simulink model "Task_No6"  (R2023b)
settings: Solver=ode5  StartTime=0.0  StopTime=3600*24*7  FixedStep=1  RelTol=1e-3
InitFcn:
  | PARAMETERS;
StartFcn:
  | PARAMETERS;
values from neighbouring files (symbols this model uses):
  Conv_C_to_K = 273.15    [PARAMETERS.m]
  P_AC_AIR_FLOW = 1    [PARAMETERS.m]
  P_CP_AIR = 1012    [PARAMETERS.m]
  P_DENSITY_AIR = 1.2041    [PARAMETERS.m]
  P_DENSITY_BRICK = 2/(10^-3)    (= 2000)    [PARAMETERS.m]
  P_DENSITY_PUR = 150    [PARAMETERS.m]
  P_EM_GLASS = 0.94    [PARAMETERS.m]
  P_EM_WALL = 0.94    [PARAMETERS.m]
  P_HANDLER_AIR_FLOW = 0.1    [PARAMETERS.m]
  P_HUMAN = 100    [PARAMETERS.m]
  P_INIT_CO2 = 420    [PARAMETERS.m]
  P_M_HUMAN_CO2 = 0.02*P_DENSITY_CO2/3600    (= 1.1e-05)    [PARAMETERS.m]
  P_M_HUMAN_VAPOR = 500*10^-3/(24*3600)    (= 5.78703703704e-06)    [PARAMETERS.m]
  P_M_WINDOW_SPEC = 20    [PARAMETERS.m]
  P_THICK_BRICK = 0.175    [PARAMETERS.m]
  P_THICK_PUR = P_THICK_WALL - P_THICK_BRICK    (= 0.125)    [PARAMETERS.m]
  RH_INIT_BDR = 40    [PARAMETERS.m]
  T_BREATH = 34    [PARAMETERS.m]
  T_COOLER = 12    [PARAMETERS.m]
  T_HEATER = 50    [PARAMETERS.m]
  T_INIT_BDR = 22    [PARAMETERS.m]
  T_INIT_OUT = 2.9    [PARAMETERS.m]
  U_WALL = 0.32    [PARAMETERS.m]
  U_WINDOW = 3.0    (= 3)    [PARAMETERS.m]
undefined symbols (not defined in the file or in its folder): P_AREA_BATH, P_AREA_BDR1, P_AREA_BDR2, P_AREA_EAST_WALL_BATH, P_AREA_EAST_WALL_BDR2, P_AREA_EAST_WALL_KIT, P_AREA_HALL, P_AREA_KIT, P_AREA_LVR, P_AREA_NORTH_WALL_BATH, P_AREA_NORTH_WALL_BDR1, P_AREA_NORTH_WALL_BDR2, P_AREA_OUTER_WALL_BATH, P_AREA_OUTER_WALL_BDR1, P_AREA_OUTER_WALL_BDR2, P_AREA_OUTER_WALL_HALL, P_AREA_OUTER_WALL_KIT, P_AREA_OUTER_WALL_LVR, P_AREA_SOUTH_WALL_KIT, P_AREA_SOUTH_WALL_LVR, P_AREA_WALL_BATH_KIT, P_AREA_WALL_BDR1_BDR2, P_AREA_WALL_BDR1_HALL, P_AREA_WALL_BDR2_BATH, P_AREA_WALL_BDR2_HALL, P_AREA_WALL_HALL_BATH, P_AREA_WALL_HALL_LVR, P_AREA_WALL_LVR_KIT, P_AREA_WIN_BATH, P_AREA_WIN_BDRS, P_AREA_WIN_KIT, P_AREA_WIN_LVR, P_M_AIR_BATH, P_M_AIR_BDR1, P_M_AIR_BDR2, P_M_AIR_HALL, P_M_AIR_KIT, P_M_AIR_LVR, TBL_SOL_EAST_01, TBL_SOL_EAST_02, TBL_SOL_EAST_03, TBL_SOL_EAST_04, TBL_SOL_EAST_05, TBL_SOL_EAST_06, TBL_SOL_EAST_07, TBL_SOL_EAST_08, TBL_SOL_EAST_09, TBL_SOL_EAST_10, TBL_SOL_EAST_11, TBL_SOL_EAST_12, TBL_SOL_NORTH_01, TBL_SOL_NORTH_02, TBL_SOL_NORTH_03, TBL_SOL_NORTH_04, TBL_SOL_NORTH_05, TBL_SOL_NORTH_06, TBL_SOL_NORTH_07, TBL_SOL_NORTH_08, TBL_SOL_NORTH_09, TBL_SOL_NORTH_10 ... (+7)
libraries: fl_lib x166, nesl_utility x88, slpidlib x3
(part 4 of 5)

== system Task_No6/sub_House/Bedroom 2/Bedroom 2/Window (BDR2<->Outside) ==
  InAir-Window : fl_lib/Thermal/Thermal Elements/Thermal Resistance  resistance=1/(U_WINDOW*P_AREA_WIN_BDRS*2)/2 K/W  T_specify=off  T_priority=None  T=0 K  T_nominal_specify=off  T_nominal_unit=K  T_nominal_value=1  Q_specify=off  Q_priority=None  Q=0 W  Q_nominal_specify=off  Q_nominal_unit=W  Q_nominal_value=1
  Thermal Mass of window : fl_lib/Thermal/Thermal Elements/Thermal Mass  mass_type=foundation.enum.constant_variable.constant  mass=P_M_WINDOW_SPEC*P_AREA_WIN_BDRS*2 kg  sp_heat=P_CP_GLASS J/(K*kg)  mass_min=1e-6 kg  num_ports=foundation.enum.numPorts2.one  m_specify=off  m_priority=High  m=1 kg  m_nominal_specify=off  m_nominal_unit=kg  m_nominal_value=1  T_specify=on  T_priority=High  T=T_INIT_BDR degC  T_nominal_specify=off  T_nominal_unit=K  T_nominal_value=1  Q_specify=off  Q_priority=None  Q=0 W  Q_nominal_specify=off  Q_nominal_unit=W  Q_nominal_value=1
  Window-OutAir : fl_lib/Thermal/Thermal Elements/Thermal Resistance  resistance=1/(U_WINDOW*P_AREA_WIN_BDRS*2)/2 K/W  T_specify=off  T_priority=None  T=0 K  T_nominal_specify=off  T_nominal_unit=K  T_nominal_value=1  Q_specify=off  Q_priority=None  Q=0 W  Q_nominal_specify=off  Q_nominal_unit=W  Q_nominal_value=1
  Conn1 : PMIOPort  Side=Right
  Conn2 : PMIOPort  Port=2  Side=Left
  Conn3 : PMIOPort  Port=3  Side=Right
  connections:
  Conn2/RConn1 -- InAir-Window/LConn1
  Conn1/RConn1 -- Window-OutAir/RConn1
  InAir-Window/RConn1 -- Thermal Mass of window/LConn1 -- Conn3/RConn1 -- Window-OutAir/LConn1

== system Task_No6/sub_House/Bedroom 2/MA Bedroom 2/Environment_in ==
  Constant1 : Constant  Value=P_INIT_CO2
  Constant4 : Constant  Value=1e5
  Constant6 : Constant  Value=Conv_C_to_K
  Controlled Reservoir (MA) : fl_lib/Moist Air/Elements/Controlled Reservoir (MA)  moisture_spec=foundation.enum.moistureSpec.RelativeHumidity  trace_gas_spec=foundation.enum.trace_gas_spec.mass_fraction  RH_ws=1  area_A=P_AREA_DUCT m^2  input_error_spec=foundation.enum.input_range_error.warn
      settings: InternalSimscapePortConfiguration="{\"Bottom\":[],\"Left\":[{\"id\":\"A\",\"label\":\"A\",\"type\":\"foundation.moist_air.moist_air\"}],\"Right\":[{\"id\":\"T\",\"label\":\"T\",\"type\":\"input\"},{\"id\":\"P\",\"label\":\"P\",\"type\":\"input\"},{\"id\":\"W\",\"label\":\"W\",\"type\":\"input\"},{\"id\":\"G\",\"label\":\"G\",\"type\":\"input\"}],\"Top\":[]}"
  Gain : Gain  Gain=1/100
  Gain2 : Gain  Gain=1e-6
  Simulink-PS Converter{3,5..7} (4 alike) : nesl_utility/Simulink-PS Converter  PhysicalDomain=network_engine_domain  SubClassName=ps_input  LeftPortType=input  RightPortType=output  PseudoPeriodic=off  Frequencies=[]  NoiseDistribution=none  NoiseParameters=[]  Unit=1  AffineConversion=off  FilteringAndDerivatives=provide  SimscapeFilterOrder=1  InputFilterTimeConstant=0.001  UdotUserProvided=0
  Sum2 : Sum  Inputs=|++
  Conn1 : PMIOPort  Side=Left
  wires:
  Constant1/1 -> Gain2/1
  Constant6/1 -> Sum2/2
  Gain/1 -> Simulink-PS Converter6/1
  Constant4/1 -> Simulink-PS Converter5/1
  Gain2/1 -> Simulink-PS Converter7/1
  Sum2/1 -> Simulink-PS Converter3/1
  [T_OUT] -> Sum2/1
  [RH_OUT] -> Gain/1
  connections:
  Simulink-PS Converter3/RConn1 -- Controlled Reservoir (MA)/RConn1
  Simulink-PS Converter7/RConn1 -- Controlled Reservoir (MA)/RConn4
  Controlled Reservoir (MA)/LConn1 -- Conn1/RConn1
  Simulink-PS Converter5/RConn1 -- Controlled Reservoir (MA)/RConn2
  Simulink-PS Converter6/RConn1 -- Controlled Reservoir (MA)/RConn3

== system Task_No6/sub_House/Bedroom 2/MA Bedroom 2/Moisture & CO2 Gain ==
  Constant : Constant  Value=T_BREATH
  Constant1 : Constant  Value=P_M_HUMAN_VAPOR
  Constant2 : Constant  Value=P_M_HUMAN_CO2
  Constant3 : Constant  Value=Conv_C_to_K
  Inhabitant CO2 Gain : fl_lib/Moist Air/Sources/Moisture & Trace Gas Sources/Trace Gas Source (MA)  source_type=foundation.enum.constant_controlled.controlled  trace_gas_mass_flow=P_M_HUMAN_CO2 kg/s  temperature_spec=foundation.enum.temperature_spec.specified  trace_gas_temperature=T_BREATH degC  Phi_S_specify=off  Phi_S_priority=None  Phi_S=0 kW  Phi_S_nominal_specify=off  Phi_S_nominal_unit=kW  Phi_S_nominal_value=1  mdot_g_S_specify=off  mdot_g_S_priority=None  mdot_g_S=0 kg/s  mdot_g_S_nominal_specify=off  mdot_g_S_nominal_unit=kg/s  mdot_g_S_nominal_value=1
      settings: InternalSimscapePortConfiguration="{\"Bottom\":[],\"Left\":[{\"id\":\"S\",\"label\":\"S\",\"type\":\"foundation.moist_air.moist_air_source\"}],\"Right\":[{\"id\":\"M\",\"label\":\"M\",\"type\":\"input\"},{\"id\":\"T\",\"label\":\"T\",\"type\":\"input\"}],\"Top\":[]}"
  Inhabitant Moisture Gain : fl_lib/Moist Air/Sources/Moisture & Trace Gas Sources/Moisture Source (MA)  source_type=foundation.enum.constant_controlled.controlled  moisture_source_spec=foundation.enum.moisture_source_spec.vapor  moisture_mass_flow=P_M_HUMAN_VAPOR kg/s  temperature_spec=foundation.enum.temperature_spec.specified  moisture_temperature=T_BREATH degC  Phi_S_specify=off  Phi_S_priority=None  Phi_S=0 kW  Phi_S_nominal_specify=off  Phi_S_nominal_unit=kW  Phi_S_nominal_value=1  mdot_w_S_specify=off  mdot_w_S_priority=None  mdot_w_S=0 kg/s  mdot_w_S_nominal_specify=off  mdot_w_S_nominal_unit=kg/s  mdot_w_S_nominal_value=1
      settings: InternalSimscapePortConfiguration="{\"Bottom\":[],\"Left\":[{\"id\":\"S\",\"label\":\"S\",\"type\":\"foundation.moist_air.moist_air_source\"}],\"Right\":[{\"id\":\"M\",\"label\":\"M\",\"type\":\"input\"},{\"id\":\"T\",\"label\":\"T\",\"type\":\"input\"}],\"Top\":[]}"
  Product : Product
  Product1 : Product
  Simulink-PS Converter : nesl_utility/Simulink-PS Converter  PhysicalDomain=network_engine_domain  SubClassName=ps_input  LeftPortType=input  RightPortType=output  PseudoPeriodic=off  Frequencies=[]  NoiseDistribution=none  NoiseParameters=[]  Unit=1  AffineConversion=off  FilteringAndDerivatives=provide  SimscapeFilterOrder=1  InputFilterTimeConstant=0.001  UdotUserProvided=0
  Simulink-PS Converter1 : nesl_utility/Simulink-PS Converter  PhysicalDomain=network_engine_domain  SubClassName=ps_input  LeftPortType=input  RightPortType=output  PseudoPeriodic=off  Frequencies=[]  NoiseDistribution=none  NoiseParameters=[]  Unit=1  AffineConversion=off  FilteringAndDerivatives=provide  SimscapeFilterOrder=1  InputFilterTimeConstant=0.001  UdotUserProvided=0
  Simulink-PS Converter3 : nesl_utility/Simulink-PS Converter  PhysicalDomain=network_engine_domain  SubClassName=ps_input  LeftPortType=input  RightPortType=output  PseudoPeriodic=off  Frequencies=[]  NoiseDistribution=none  NoiseParameters=[]  Unit=1  AffineConversion=off  FilteringAndDerivatives=provide  SimscapeFilterOrder=1  InputFilterTimeConstant=0.001  UdotUserProvided=0
  Sum : Sum  Inputs=++|
  Conn1 : PMIOPort  Side=Left
  wires:
  Sum/1 -> Simulink-PS Converter1/1
  Product1/1 -> Simulink-PS Converter3/1
  Constant1/1 -> Product/2
  Constant/1 -> Sum/2
  Constant3/1 -> Sum/1
  [N_BDR2] -> Product/1
  Product/1 -> Simulink-PS Converter/1
  Constant2/1 -> Product1/2
  [N_BDR2] -> Product1/1
  connections:
  Simulink-PS Converter/RConn1 -- Inhabitant Moisture Gain/RConn1
  Simulink-PS Converter3/RConn1 -- Inhabitant CO2 Gain/RConn1
  Conn1/RConn1 -- Inhabitant Moisture Gain/LConn1 -- Inhabitant CO2 Gain/LConn1
  Inhabitant CO2 Gain/RConn2 -- Simulink-PS Converter1/RConn1 -- Inhabitant Moisture Gain/RConn2

== system Task_No6/sub_House/Hallway/Hallway/Ceiling & Floor (Hall<->Above & Below) ==
  Ceiling-InAir : fl_lib/Thermal/Thermal Elements/Thermal Resistance  resistance=1/(U_CEIL*P_AREA_HALL) K/W  T_specify=off  T_priority=None  T=0 K  T_nominal_specify=off  T_nominal_unit=K  T_nominal_value=1  Q_specify=off  Q_priority=None  Q=0 W  Q_nominal_specify=off  Q_nominal_unit=W  Q_nominal_value=1
  Floor-InAir : fl_lib/Thermal/Thermal Elements/Thermal Resistance  resistance=1/(U_CEIL*P_AREA_HALL) K/W  T_specify=off  T_priority=None  T=0 K  T_nominal_specify=off  T_nominal_unit=K  T_nominal_value=1  Q_specify=off  Q_priority=None  Q=0 W  Q_nominal_specify=off  Q_nominal_unit=W  Q_nominal_value=1
  Conn1 : PMIOPort  Side=Left
  Conn2 : PMIOPort  Port=2  Side=Right
  connections:
  Floor-InAir/RConn1 -- Ceiling-InAir/RConn1 -- Conn2/RConn1
  Floor-InAir/LConn1 -- Ceiling-InAir/LConn1 -- Conn1/RConn1

== system Task_No6/sub_House/Hallway/Hallway/Inside Enivornment Temperature ==
  T_ENV : Inport
  Constant2 : Constant  Value=Conv_C_to_K
  Controlled Temperature Source : fl_lib/Thermal/Thermal Sources/Controlled Temperature Source
  Simulink-PS Converter1 : nesl_utility/Simulink-PS Converter  PhysicalDomain=network_engine_domain  SubClassName=ps_input  LeftPortType=input  RightPortType=output  PseudoPeriodic=off  Frequencies=[]  NoiseDistribution=none  NoiseParameters=[]  Unit=1  AffineConversion=off  FilteringAndDerivatives=provide  SimscapeFilterOrder=1  InputFilterTimeConstant=0.001  UdotUserProvided=0
  Sum : Sum  Inputs=|++
  Thermal Reference1 : fl_lib/Thermal/Thermal Elements/Thermal Reference
  Conn1 : PMIOPort  Side=Left
  wires:
  T_ENV/1 -> Sum/1
  Constant2/1 -> Sum/2
  Sum/1 -> Simulink-PS Converter1/1
  connections:
  Controlled Temperature Source/LConn1 -- Conn1/RConn1
  Simulink-PS Converter1/RConn1 -- Controlled Temperature Source/RConn1
  Thermal Reference1/LConn1 -- Controlled Temperature Source/RConn2

== system Task_No6/sub_House/Hallway/Hallway/Outside Temperature ==
  T_OUT : Inport
  Constant2 : Constant  Value=Conv_C_to_K
  Controlled Temperature Source : fl_lib/Thermal/Thermal Sources/Controlled Temperature Source
  Simulink-PS Converter1 : nesl_utility/Simulink-PS Converter  PhysicalDomain=network_engine_domain  SubClassName=ps_input  LeftPortType=input  RightPortType=output  PseudoPeriodic=off  Frequencies=[]  NoiseDistribution=none  NoiseParameters=[]  Unit=1  AffineConversion=off  FilteringAndDerivatives=provide  SimscapeFilterOrder=1  InputFilterTimeConstant=0.001  UdotUserProvided=0
  Sum : Sum  Inputs=|++
  Thermal Reference1 : fl_lib/Thermal/Thermal Elements/Thermal Reference
  Conn1 : PMIOPort  Side=Left
  wires:
  Sum/1 -> Simulink-PS Converter1/1
  Constant2/1 -> Sum/2
  T_OUT/1 -> Sum/1
  connections:
  Thermal Reference1/LConn1 -- Controlled Temperature Source/RConn2
  Simulink-PS Converter1/RConn1 -- Controlled Temperature Source/RConn1
  Controlled Temperature Source/LConn1 -- Conn1/RConn1

== system Task_No6/sub_House/Hallway/Hallway/TEMP_01 ==
  Constant2 : Constant  Value=Conv_C_to_K
  PS-Simulink Converter : nesl_utility/PS-Simulink Converter  PhysicalDomain=network_engine_domain  SubClassName=ps_output  LeftPortType=input  RightPortType=output  PseudoPeriodic=off  Frequencies=[]  VectorFormat=inherit  Unit=inherit  AffineConversion=off
  Sum : Sum  Inputs=|+-
  Temperature Sensor : fl_lib/Thermal/Thermal Sensors/Temperature Sensor  temperature_measure=foundation.enum.MeasurementReference.difference
  Thermal Reference2 : fl_lib/Thermal/Thermal Elements/Thermal Reference
  PS : PMIOPort  Side=Left
  Sim : Outport
  wires:
  Sum/1 -> Sim/1
  PS-Simulink Converter/1 -> Sum/1
  Constant2/1 -> Sum/2
  connections:
  Thermal Reference2/LConn1 -- Temperature Sensor/RConn1
  PS-Simulink Converter/LConn1 -- Temperature Sensor/RConn2
  PS/RConn1 -- Temperature Sensor/LConn1

== system Task_No6/sub_House/Hallway/Hallway/Wall (Hall<->Outside) ==
  InAir-Wall : fl_lib/Thermal/Thermal Elements/Thermal Resistance  resistance=1/(U_WALL*P_AREA_OUTER_WALL_HALL)/2 K/W  T_specify=off  T_priority=None  T=0 K  T_nominal_specify=off  T_nominal_unit=K  T_nominal_value=1  Q_specify=off  Q_priority=None  Q=0 W  Q_nominal_specify=off  Q_nominal_unit=W  Q_nominal_value=1
  Thermal Mass of wall : fl_lib/Thermal/Thermal Elements/Thermal Mass  mass_type=foundation.enum.constant_variable.constant  mass=P_AREA_OUTER_WALL_HALL*(P_THICK_BRICK*P_DENSITY_BRICK+P_THICK_PUR*P_DENSITY_PUR) kg  sp_heat=P_CP_WALL J/(K*kg)  mass_min=1e-6 kg  num_ports=foundation.enum.numPorts2.one  m_specify=off  m_priority=High  m=1 kg  m_nominal_specify=off  m_nominal_unit=kg  m_nominal_value=1  T_specify=on  T_priority=High  T=T_INIT_BDR degC  T_nominal_specify=off  T_nominal_unit=K  T_nominal_value=1  Q_specify=off  Q_priority=None  Q=0 W  Q_nominal_specify=off  Q_nominal_unit=W  Q_nominal_value=1
  Wall-OutAir : fl_lib/Thermal/Thermal Elements/Thermal Resistance  resistance=1/(U_WALL*P_AREA_OUTER_WALL_HALL)/2 K/W  T_specify=off  T_priority=None  T=0 K  T_nominal_specify=off  T_nominal_unit=K  T_nominal_value=1  Q_specify=off  Q_priority=None  Q=0 W  Q_nominal_specify=off  Q_nominal_unit=W  Q_nominal_value=1
  Conn1 : PMIOPort  Side=Left
  Conn2 : PMIOPort  Port=2  Side=Right
  connections:
  Conn1/RConn1 -- InAir-Wall/LConn1
  InAir-Wall/RConn1 -- Thermal Mass of wall/LConn1 -- Wall-OutAir/LConn1
  Wall-OutAir/RConn1 -- Conn2/RConn1

== system Task_No6/sub_House/Kitchen/Kitchen/Ceiling & Floor (KIT<->Above & Below) ==
  Ceiling-InAir : fl_lib/Thermal/Thermal Elements/Thermal Resistance  resistance=1/(U_CEIL*P_AREA_KIT) K/W  T_specify=off  T_priority=None  T=0 K  T_nominal_specify=off  T_nominal_unit=K  T_nominal_value=1  Q_specify=off  Q_priority=None  Q=0 W  Q_nominal_specify=off  Q_nominal_unit=W  Q_nominal_value=1
  Floor-InAir : fl_lib/Thermal/Thermal Elements/Thermal Resistance  resistance=1/(U_CEIL*P_AREA_KIT) K/W  T_specify=off  T_priority=None  T=0 K  T_nominal_specify=off  T_nominal_unit=K  T_nominal_value=1  Q_specify=off  Q_priority=None  Q=0 W  Q_nominal_specify=off  Q_nominal_unit=W  Q_nominal_value=1
  Conn1 : PMIOPort  Side=Left
  Conn2 : PMIOPort  Port=2  Side=Right
  connections:
  Floor-InAir/RConn1 -- Ceiling-InAir/RConn1 -- Conn2/RConn1
  Floor-InAir/LConn1 -- Ceiling-InAir/LConn1 -- Conn1/RConn1

== system Task_No6/sub_House/Kitchen/Kitchen/Heat source human ==
  Constant : Constant  Value=P_HUMAN
  Controlled Heat Flow Rate Source : fl_lib/Thermal/Thermal Sources/Controlled Heat Flow Rate Source
  Product : Product
  Simulink-PS Converter : nesl_utility/Simulink-PS Converter  PhysicalDomain=network_engine_domain  SubClassName=ps_input  LeftPortType=input  RightPortType=output  PseudoPeriodic=off  Frequencies=[]  NoiseDistribution=none  NoiseParameters=[]  Unit=1  AffineConversion=off  FilteringAndDerivatives=provide  SimscapeFilterOrder=1  InputFilterTimeConstant=0.001  UdotUserProvided=0
  Thermal Reference : fl_lib/Thermal/Thermal Elements/Thermal Reference
  Conn1 : PMIOPort  Side=Left
  wires:
  [N_KIT] -> Product/1
  Constant/1 -> Product/2
  Product/1 -> Simulink-PS Converter/1
  connections:
  Thermal Reference/LConn1 -- Controlled Heat Flow Rate Source/RConn2
  Simulink-PS Converter/RConn1 -- Controlled Heat Flow Rate Source/RConn1
  Controlled Heat Flow Rate Source/LConn1 -- Conn1/RConn1

== system Task_No6/sub_House/Kitchen/Kitchen/Inside Enivornment Temperature ==
  T_ENV : Inport
  Constant2 : Constant  Value=Conv_C_to_K
  Controlled Temperature Source : fl_lib/Thermal/Thermal Sources/Controlled Temperature Source
  Simulink-PS Converter1 : nesl_utility/Simulink-PS Converter  PhysicalDomain=network_engine_domain  SubClassName=ps_input  LeftPortType=input  RightPortType=output  PseudoPeriodic=off  Frequencies=[]  NoiseDistribution=none  NoiseParameters=[]  Unit=1  AffineConversion=off  FilteringAndDerivatives=provide  SimscapeFilterOrder=1  InputFilterTimeConstant=0.001  UdotUserProvided=0
  Sum : Sum  Inputs=|++
  Thermal Reference1 : fl_lib/Thermal/Thermal Elements/Thermal Reference
  Conn1 : PMIOPort  Side=Left
  wires:
  T_ENV/1 -> Sum/1
  Constant2/1 -> Sum/2
  Sum/1 -> Simulink-PS Converter1/1
  connections:
  Controlled Temperature Source/LConn1 -- Conn1/RConn1
  Simulink-PS Converter1/RConn1 -- Controlled Temperature Source/RConn1
  Thermal Reference1/LConn1 -- Controlled Temperature Source/RConn2

== system Task_No6/sub_House/Kitchen/Kitchen/Outside Temperature ==
  T_OUT : Inport
  Constant2 : Constant  Value=Conv_C_to_K
  Controlled Temperature Source : fl_lib/Thermal/Thermal Sources/Controlled Temperature Source
  Simulink-PS Converter1 : nesl_utility/Simulink-PS Converter  PhysicalDomain=network_engine_domain  SubClassName=ps_input  LeftPortType=input  RightPortType=output  PseudoPeriodic=off  Frequencies=[]  NoiseDistribution=none  NoiseParameters=[]  Unit=1  AffineConversion=off  FilteringAndDerivatives=provide  SimscapeFilterOrder=1  InputFilterTimeConstant=0.001  UdotUserProvided=0
  Sum : Sum  Inputs=|++
  Thermal Reference1 : fl_lib/Thermal/Thermal Elements/Thermal Reference
  Conn1 : PMIOPort  Side=Left
  wires:
  Sum/1 -> Simulink-PS Converter1/1
  Constant2/1 -> Sum/2
  T_OUT/1 -> Sum/1
  connections:
  Thermal Reference1/LConn1 -- Controlled Temperature Source/RConn2
  Simulink-PS Converter1/RConn1 -- Controlled Temperature Source/RConn1
  Controlled Temperature Source/LConn1 -- Conn1/RConn1

== system Task_No6/sub_House/Kitchen/Kitchen/SOLAR__WALL ==
  Add : Sum
  Constant : Constant  Value=P_AREA_EAST_WALL_KIT
  Constant1 : Constant  Value=P_EM_WALL
  Constant2 : Constant  Value=P_AREA_SOUTH_WALL_KIT
  Constant3 : Constant  Value=P_EM_WALL
  Controlled Heat Flow Rate Source : fl_lib/Thermal/Thermal Sources/Controlled Heat Flow Rate Source
  Product : Product  Inputs=3
  Product1 : Product  Inputs=3
  Simulink-PS Converter : nesl_utility/Simulink-PS Converter  PhysicalDomain=network_engine_domain  SubClassName=ps_input  LeftPortType=input  RightPortType=output  PseudoPeriodic=off  Frequencies=[]  NoiseDistribution=none  NoiseParameters=[]  Unit=1  AffineConversion=off  FilteringAndDerivatives=provide  SimscapeFilterOrder=1  InputFilterTimeConstant=0.001  UdotUserProvided=0
  Thermal Reference : fl_lib/Thermal/Thermal Elements/Thermal Reference
  Conn1 : PMIOPort  Side=Left
  wires:
  Constant/1 -> Product/2
  Constant1/1 -> Product/1
  [SOL_EAST] -> Product/3
  Product/1 -> Add/1
  Constant3/1 -> Product1/1
  [SOL_SOUTH] -> Product1/3
  Constant2/1 -> Product1/2
  Add/1 -> Simulink-PS Converter/1
  Product1/1 -> Add/2
  connections:
  Controlled Heat Flow Rate Source/LConn1 -- Conn1/RConn1
  Simulink-PS Converter/RConn1 -- Controlled Heat Flow Rate Source/RConn1
  Thermal Reference/LConn1 -- Controlled Heat Flow Rate Source/RConn2

== system Task_No6/sub_House/Kitchen/Kitchen/SOLAR__WINDOW ==
  Constant : Constant  Value=P_AREA_WIN_KIT
  Constant1 : Constant  Value=P_EM_GLASS
  Controlled Heat Flow Rate Source : fl_lib/Thermal/Thermal Sources/Controlled Heat Flow Rate Source
  Product : Product  Inputs=3
  Simulink-PS Converter : nesl_utility/Simulink-PS Converter  PhysicalDomain=network_engine_domain  SubClassName=ps_input  LeftPortType=input  RightPortType=output  PseudoPeriodic=off  Frequencies=[]  NoiseDistribution=none  NoiseParameters=[]  Unit=1  AffineConversion=off  FilteringAndDerivatives=provide  SimscapeFilterOrder=1  InputFilterTimeConstant=0.001  UdotUserProvided=0
  Thermal Reference : fl_lib/Thermal/Thermal Elements/Thermal Reference
  Conn1 : PMIOPort  Side=Left
  wires:
  Product/1 -> Simulink-PS Converter/1
  [SOL_SOUTH] -> Product/3
  Constant1/1 -> Product/1
  Constant/1 -> Product/2
  connections:
  Thermal Reference/LConn1 -- Controlled Heat Flow Rate Source/RConn2
  Simulink-PS Converter/RConn1 -- Controlled Heat Flow Rate Source/RConn1
  Controlled Heat Flow Rate Source/LConn1 -- Conn1/RConn1

== system Task_No6/sub_House/Kitchen/Kitchen/TEMP_01 ==
  Constant2 : Constant  Value=Conv_C_to_K
  PS-Simulink Converter : nesl_utility/PS-Simulink Converter  PhysicalDomain=network_engine_domain  SubClassName=ps_output  LeftPortType=input  RightPortType=output  PseudoPeriodic=off  Frequencies=[]  VectorFormat=inherit  Unit=inherit  AffineConversion=off
  Sum : Sum  Inputs=|+-
  Temperature Sensor : fl_lib/Thermal/Thermal Sensors/Temperature Sensor  temperature_measure=foundation.enum.MeasurementReference.difference
  Thermal Reference2 : fl_lib/Thermal/Thermal Elements/Thermal Reference
  PS : PMIOPort  Side=Left
  Sim : Outport
  wires:
  Sum/1 -> Sim/1
  PS-Simulink Converter/1 -> Sum/1
  Constant2/1 -> Sum/2
  connections:
  Thermal Reference2/LConn1 -- Temperature Sensor/RConn1
  PS-Simulink Converter/LConn1 -- Temperature Sensor/RConn2
  PS/RConn1 -- Temperature Sensor/LConn1

== system Task_No6/sub_House/Kitchen/Kitchen/Wall (KIT<->Outside) ==
  InAir-Wall : fl_lib/Thermal/Thermal Elements/Thermal Resistance  resistance=1/(U_WALL*P_AREA_OUTER_WALL_KIT)/2 K/W  T_specify=off  T_priority=None  T=0 K  T_nominal_specify=off  T_nominal_unit=K  T_nominal_value=1  Q_specify=off  Q_priority=None  Q=0 W  Q_nominal_specify=off  Q_nominal_unit=W  Q_nominal_value=1
  Thermal Mass of wall : fl_lib/Thermal/Thermal Elements/Thermal Mass  mass_type=foundation.enum.constant_variable.constant  mass=P_AREA_OUTER_WALL_KIT*(P_THICK_BRICK*P_DENSITY_BRICK+P_THICK_PUR*P_DENSITY_PUR) kg  sp_heat=P_CP_WALL J/(K*kg)  mass_min=1e-6 kg  num_ports=foundation.enum.numPorts2.one  m_specify=off  m_priority=High  m=1 kg  m_nominal_specify=off  m_nominal_unit=kg  m_nominal_value=1  T_specify=on  T_priority=High  T=T_INIT_BDR degC  T_nominal_specify=off  T_nominal_unit=K  T_nominal_value=1  Q_specify=off  Q_priority=None  Q=0 W  Q_nominal_specify=off  Q_nominal_unit=W  Q_nominal_value=1
  Wall-OutAir : fl_lib/Thermal/Thermal Elements/Thermal Resistance  resistance=1/(U_WALL*P_AREA_OUTER_WALL_KIT)/2 K/W  T_specify=off  T_priority=None  T=0 K  T_nominal_specify=off  T_nominal_unit=K  T_nominal_value=1  Q_specify=off  Q_priority=None  Q=0 W  Q_nominal_specify=off  Q_nominal_unit=W  Q_nominal_value=1
  Conn1 : PMIOPort  Side=Left
  Conn3 : PMIOPort  Port=2  Side=Right
  Conn2 : PMIOPort  Port=3  Side=Right
  connections:
  Conn1/RConn1 -- InAir-Wall/LConn1
  InAir-Wall/RConn1 -- Conn3/RConn1 -- Thermal Mass of wall/LConn1 -- Wall-OutAir/LConn1
  Wall-OutAir/RConn1 -- Conn2/RConn1

== system Task_No6/sub_House/Kitchen/Kitchen/Window (KIT<->Outside) ==
  InAir-Window : fl_lib/Thermal/Thermal Elements/Thermal Resistance  resistance=1/(U_WINDOW*P_AREA_WIN_KIT)/2 K/W  T_specify=off  T_priority=None  T=0 K  T_nominal_specify=off  T_nominal_unit=K  T_nominal_value=1  Q_specify=off  Q_priority=None  Q=0 W  Q_nominal_specify=off  Q_nominal_unit=W  Q_nominal_value=1
  Thermal Mass of window : fl_lib/Thermal/Thermal Elements/Thermal Mass  mass_type=foundation.enum.constant_variable.constant  mass=P_M_WINDOW_SPEC*P_AREA_WIN_KIT kg  sp_heat=P_CP_GLASS J/(K*kg)  mass_min=1e-6 kg  num_ports=foundation.enum.numPorts2.one  m_specify=off  m_priority=High  m=1 kg  m_nominal_specify=off  m_nominal_unit=kg  m_nominal_value=1  T_specify=on  T_priority=High  T=T_INIT_BDR degC  T_nominal_specify=off  T_nominal_unit=K  T_nominal_value=1  Q_specify=off  Q_priority=None  Q=0 W  Q_nominal_specify=off  Q_nominal_unit=W  Q_nominal_value=1
  Window-OutAir : fl_lib/Thermal/Thermal Elements/Thermal Resistance  resistance=1/(U_WINDOW*P_AREA_WIN_KIT)/2 K/W  T_specify=off  T_priority=None  T=0 K  T_nominal_specify=off  T_nominal_unit=K  T_nominal_value=1  Q_specify=off  Q_priority=None  Q=0 W  Q_nominal_specify=off  Q_nominal_unit=W  Q_nominal_value=1
  Conn1 : PMIOPort  Side=Right
  Conn2 : PMIOPort  Port=2  Side=Left
  Conn3 : PMIOPort  Port=3  Side=Right
  connections:
  Thermal Mass of window/LConn1 -- Conn3/RConn1 -- Window-OutAir/LConn1 -- InAir-Window/RConn1
  Conn1/RConn1 -- Window-OutAir/RConn1
  Conn2/RConn1 -- InAir-Window/LConn1

== system Task_No6/sub_House/Kitchen/MA Kitchen/Environment_out ==
  Constant1 : Constant  Value=P_INIT_CO2
  Constant4 : Constant  Value=1e5
  Constant6 : Constant  Value=Conv_C_to_K
  Controlled Reservoir (MA) : fl_lib/Moist Air/Elements/Controlled Reservoir (MA)  moisture_spec=foundation.enum.moistureSpec.RelativeHumidity  trace_gas_spec=foundation.enum.trace_gas_spec.mass_fraction  RH_ws=1  area_A=P_AREA_DUCT m^2  input_error_spec=foundation.enum.input_range_error.warn
      settings: InternalSimscapePortConfiguration="{\"Bottom\":[],\"Left\":[{\"id\":\"A\",\"label\":\"A\",\"type\":\"foundation.moist_air.moist_air\"}],\"Right\":[{\"id\":\"T\",\"label\":\"T\",\"type\":\"input\"},{\"id\":\"P\",\"label\":\"P\",\"type\":\"input\"},{\"id\":\"W\",\"label\":\"W\",\"type\":\"input\"},{\"id\":\"G\",\"label\":\"G\",\"type\":\"input\"}],\"Top\":[]}"
  Gain : Gain  Gain=1/100
  Gain2 : Gain  Gain=1e-6
  Simulink-PS Converter{3,5..7} (4 alike) : nesl_utility/Simulink-PS Converter  PhysicalDomain=network_engine_domain  SubClassName=ps_input  LeftPortType=input  RightPortType=output  PseudoPeriodic=off  Frequencies=[]  NoiseDistribution=none  NoiseParameters=[]  Unit=1  AffineConversion=off  FilteringAndDerivatives=provide  SimscapeFilterOrder=1  InputFilterTimeConstant=0.001  UdotUserProvided=0
  Sum2 : Sum  Inputs=|++
  Conn1 : PMIOPort  Side=Left
  wires:
  [RH_OUT] -> Gain/1
  [T_OUT] -> Sum2/1
  Sum2/1 -> Simulink-PS Converter3/1
  Gain2/1 -> Simulink-PS Converter7/1
  Constant4/1 -> Simulink-PS Converter5/1
  Gain/1 -> Simulink-PS Converter6/1
  Constant6/1 -> Sum2/2
  Constant1/1 -> Gain2/1
  connections:
  Simulink-PS Converter6/RConn1 -- Controlled Reservoir (MA)/RConn3
  Simulink-PS Converter5/RConn1 -- Controlled Reservoir (MA)/RConn2
  Controlled Reservoir (MA)/LConn1 -- Conn1/RConn1
  Simulink-PS Converter7/RConn1 -- Controlled Reservoir (MA)/RConn4
  Simulink-PS Converter3/RConn1 -- Controlled Reservoir (MA)/RConn1

== system Task_No6/sub_House/Kitchen/MA Kitchen/Moisture & CO2 Gain ==
  Constant : Constant  Value=T_BREATH
  Constant1 : Constant  Value=P_M_HUMAN_VAPOR
  Constant2 : Constant  Value=P_M_HUMAN_CO2
  Constant3 : Constant  Value=Conv_C_to_K
  Inhabitant CO2 Gain : fl_lib/Moist Air/Sources/Moisture & Trace Gas Sources/Trace Gas Source (MA)  source_type=foundation.enum.constant_controlled.controlled  trace_gas_mass_flow=P_M_HUMAN_CO2 kg/s  temperature_spec=foundation.enum.temperature_spec.specified  trace_gas_temperature=T_BREATH degC  Phi_S_specify=off  Phi_S_priority=None  Phi_S=0 kW  Phi_S_nominal_specify=off  Phi_S_nominal_unit=kW  Phi_S_nominal_value=1  mdot_g_S_specify=off  mdot_g_S_priority=None  mdot_g_S=0 kg/s  mdot_g_S_nominal_specify=off  mdot_g_S_nominal_unit=kg/s  mdot_g_S_nominal_value=1
      settings: InternalSimscapePortConfiguration="{\"Bottom\":[],\"Left\":[{\"id\":\"S\",\"label\":\"S\",\"type\":\"foundation.moist_air.moist_air_source\"}],\"Right\":[{\"id\":\"M\",\"label\":\"M\",\"type\":\"input\"},{\"id\":\"T\",\"label\":\"T\",\"type\":\"input\"}],\"Top\":[]}"
  Inhabitant Moisture Gain : fl_lib/Moist Air/Sources/Moisture & Trace Gas Sources/Moisture Source (MA)  source_type=foundation.enum.constant_controlled.controlled  moisture_source_spec=foundation.enum.moisture_source_spec.vapor  moisture_mass_flow=P_M_HUMAN_VAPOR kg/s  temperature_spec=foundation.enum.temperature_spec.specified  moisture_temperature=T_BREATH degC  Phi_S_specify=off  Phi_S_priority=None  Phi_S=0 kW  Phi_S_nominal_specify=off  Phi_S_nominal_unit=kW  Phi_S_nominal_value=1  mdot_w_S_specify=off  mdot_w_S_priority=None  mdot_w_S=0 kg/s  mdot_w_S_nominal_specify=off  mdot_w_S_nominal_unit=kg/s  mdot_w_S_nominal_value=1
      settings: InternalSimscapePortConfiguration="{\"Bottom\":[],\"Left\":[{\"id\":\"S\",\"label\":\"S\",\"type\":\"foundation.moist_air.moist_air_source\"}],\"Right\":[{\"id\":\"M\",\"label\":\"M\",\"type\":\"input\"},{\"id\":\"T\",\"label\":\"T\",\"type\":\"input\"}],\"Top\":[]}"
  Product : Product
  Product1 : Product
  Simulink-PS Converter : nesl_utility/Simulink-PS Converter  PhysicalDomain=network_engine_domain  SubClassName=ps_input  LeftPortType=input  RightPortType=output  PseudoPeriodic=off  Frequencies=[]  NoiseDistribution=none  NoiseParameters=[]  Unit=1  AffineConversion=off  FilteringAndDerivatives=provide  SimscapeFilterOrder=1  InputFilterTimeConstant=0.001  UdotUserProvided=0
  Simulink-PS Converter1 : nesl_utility/Simulink-PS Converter  PhysicalDomain=network_engine_domain  SubClassName=ps_input  LeftPortType=input  RightPortType=output  PseudoPeriodic=off  Frequencies=[]  NoiseDistribution=none  NoiseParameters=[]  Unit=1  AffineConversion=off  FilteringAndDerivatives=provide  SimscapeFilterOrder=1  InputFilterTimeConstant=0.001  UdotUserProvided=0
  Simulink-PS Converter3 : nesl_utility/Simulink-PS Converter  PhysicalDomain=network_engine_domain  SubClassName=ps_input  LeftPortType=input  RightPortType=output  PseudoPeriodic=off  Frequencies=[]  NoiseDistribution=none  NoiseParameters=[]  Unit=1  AffineConversion=off  FilteringAndDerivatives=provide  SimscapeFilterOrder=1  InputFilterTimeConstant=0.001  UdotUserProvided=0
  Sum : Sum  Inputs=++|
  Conn1 : PMIOPort  Side=Left
  wires:
  Constant3/1 -> Sum/1
  Constant/1 -> Sum/2
  Constant1/1 -> Product/2
  Constant2/1 -> Product1/2
  Sum/1 -> Simulink-PS Converter1/1
  [N_KIT] -> Product/1
  Product/1 -> Simulink-PS Converter/1
  [N_KIT] -> Product1/1
  Product1/1 -> Simulink-PS Converter3/1
  connections:
  Inhabitant Moisture Gain/RConn2 -- Simulink-PS Converter1/RConn1 -- Inhabitant CO2 Gain/RConn2
  Inhabitant CO2 Gain/LConn1 -- Inhabitant Moisture Gain/LConn1 -- Conn1/RConn1
  Simulink-PS Converter3/RConn1 -- Inhabitant CO2 Gain/RConn1
  Simulink-PS Converter/RConn1 -- Inhabitant Moisture Gain/RConn1

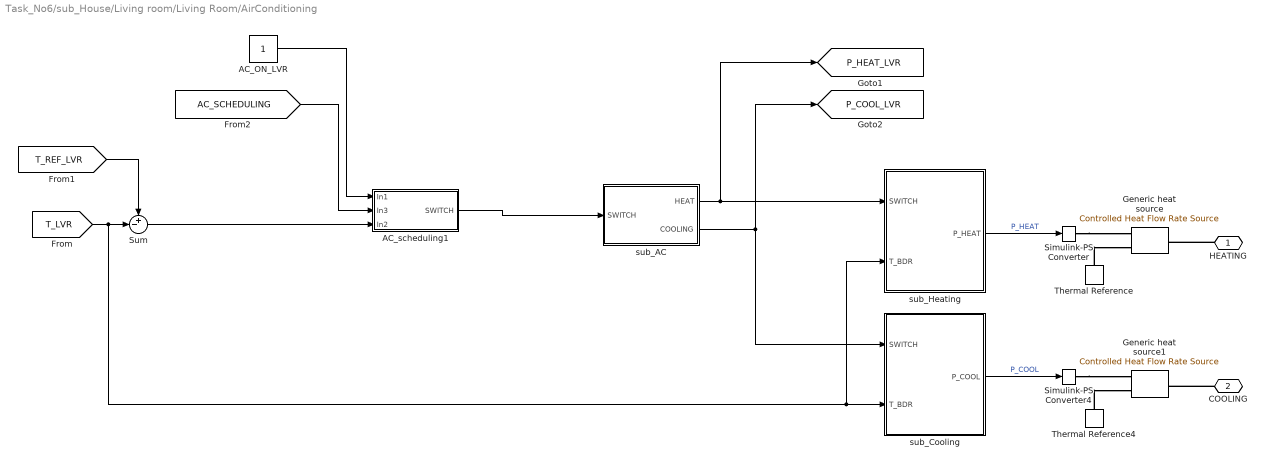
== system Task_No6/sub_House/Living room/Living Room/AirConditioning ==
  AC_ON_LVR : Constant
  AC_scheduling1 : Subsystem
  Generic heat source : fl_lib/Thermal/Thermal Sources/Controlled Heat Flow Rate Source
  Generic heat source1 : fl_lib/Thermal/Thermal Sources/Controlled Heat Flow Rate Source
  Simulink-PS Converter : nesl_utility/Simulink-PS Converter  PhysicalDomain=network_engine_domain  SubClassName=ps_input  LeftPortType=input  RightPortType=output  PseudoPeriodic=off  Frequencies=[]  NoiseDistribution=none  NoiseParameters=[]  Unit=1  AffineConversion=off  FilteringAndDerivatives=provide  SimscapeFilterOrder=1  InputFilterTimeConstant=0.001  UdotUserProvided=0
  Simulink-PS Converter4 : nesl_utility/Simulink-PS Converter  PhysicalDomain=network_engine_domain  SubClassName=ps_input  LeftPortType=input  RightPortType=output  PseudoPeriodic=off  Frequencies=[]  NoiseDistribution=none  NoiseParameters=[]  Unit=1  AffineConversion=off  FilteringAndDerivatives=provide  SimscapeFilterOrder=1  InputFilterTimeConstant=0.001  UdotUserProvided=0
  Sum : Sum  Inputs=+-|
  Thermal Reference : fl_lib/Thermal/Thermal Elements/Thermal Reference
  Thermal Reference4 : fl_lib/Thermal/Thermal Elements/Thermal Reference
  sub_AC : Subsystem
  sub_Cooling : Subsystem
  sub_Heating : Subsystem
  HEATING : PMIOPort  Side=Right
  COOLING : PMIOPort  Port=2  Side=Right
  tag scope: P_COOL_LVR=global, P_HEAT_LVR=global
  wires:
  sub_AC/2(COOLING) -> [P_COOL_LVR], sub_Cooling/1(SWITCH)
  sub_AC/1(HEAT) -> [P_HEAT_LVR], sub_Heating/1(SWITCH)
  [T_LVR] -> sub_Heating/2(T_BDR), sub_Cooling/2(T_BDR), Sum/2
  sub_Heating/1(P_HEAT) -> Simulink-PS Converter/1  "P_HEAT"
  sub_Cooling/1(P_COOL) -> Simulink-PS Converter4/1  "P_COOL"
  [T_REF_LVR] -> Sum/1
  AC_scheduling1/1(SWITCH) -> sub_AC/1(SWITCH)
  AC_ON_LVR/1 -> AC_scheduling1/1(In1)
  [AC_SCHEDULING] -> AC_scheduling1/2(In3)
  Sum/1 -> AC_scheduling1/3(In2)
  connections:
  Thermal Reference4/LConn1 -- Generic heat source1/RConn2
  Thermal Reference/LConn1 -- Generic heat source/RConn2
  Simulink-PS Converter4/RConn1 -- Generic heat source1/RConn1
  Simulink-PS Converter/RConn1 -- Generic heat source/RConn1
  HEATING/RConn1 -- Generic heat source/LConn1
  COOLING/RConn1 -- Generic heat source1/LConn1

== system Task_No6/sub_House/Living room/Living Room/Ceiling & Floor (LVR<->Above & Below) ==
  Ceiling-InAir : fl_lib/Thermal/Thermal Elements/Thermal Resistance  resistance=1/(U_CEIL*P_AREA_LVR) K/W  T_specify=off  T_priority=None  T=0 K  T_nominal_specify=off  T_nominal_unit=K  T_nominal_value=1  Q_specify=off  Q_priority=None  Q=0 W  Q_nominal_specify=off  Q_nominal_unit=W  Q_nominal_value=1
  Floor-InAir : fl_lib/Thermal/Thermal Elements/Thermal Resistance  resistance=1/(U_CEIL*P_AREA_LVR) K/W  T_specify=off  T_priority=None  T=0 K  T_nominal_specify=off  T_nominal_unit=K  T_nominal_value=1  Q_specify=off  Q_priority=None  Q=0 W  Q_nominal_specify=off  Q_nominal_unit=W  Q_nominal_value=1
  Conn1 : PMIOPort  Side=Left
  Conn2 : PMIOPort  Port=2  Side=Right
  connections:
  Conn1/RConn1 -- Ceiling-InAir/LConn1 -- Floor-InAir/LConn1
  Conn2/RConn1 -- Ceiling-InAir/RConn1 -- Floor-InAir/RConn1

== system Task_No6/sub_House/Living room/Living Room/Heat source human ==
  Constant : Constant  Value=P_HUMAN
  Controlled Heat Flow Rate Source : fl_lib/Thermal/Thermal Sources/Controlled Heat Flow Rate Source
  Product : Product
  Simulink-PS Converter : nesl_utility/Simulink-PS Converter  PhysicalDomain=network_engine_domain  SubClassName=ps_input  LeftPortType=input  RightPortType=output  PseudoPeriodic=off  Frequencies=[]  NoiseDistribution=none  NoiseParameters=[]  Unit=1  AffineConversion=off  FilteringAndDerivatives=provide  SimscapeFilterOrder=1  InputFilterTimeConstant=0.001  UdotUserProvided=0
  Thermal Reference : fl_lib/Thermal/Thermal Elements/Thermal Reference
  Conn1 : PMIOPort  Side=Left
  wires:
  [N_LVR] -> Product/1
  Constant/1 -> Product/2
  Product/1 -> Simulink-PS Converter/1
  connections:
  Thermal Reference/LConn1 -- Controlled Heat Flow Rate Source/RConn2
  Simulink-PS Converter/RConn1 -- Controlled Heat Flow Rate Source/RConn1
  Controlled Heat Flow Rate Source/LConn1 -- Conn1/RConn1

== system Task_No6/sub_House/Living room/Living Room/Inside Enivornment Temperature ==
  T_ENV : Inport
  Constant2 : Constant  Value=Conv_C_to_K
  Controlled Temperature Source : fl_lib/Thermal/Thermal Sources/Controlled Temperature Source
  Simulink-PS Converter1 : nesl_utility/Simulink-PS Converter  PhysicalDomain=network_engine_domain  SubClassName=ps_input  LeftPortType=input  RightPortType=output  PseudoPeriodic=off  Frequencies=[]  NoiseDistribution=none  NoiseParameters=[]  Unit=1  AffineConversion=off  FilteringAndDerivatives=provide  SimscapeFilterOrder=1  InputFilterTimeConstant=0.001  UdotUserProvided=0
  Sum : Sum  Inputs=|++
  Thermal Reference1 : fl_lib/Thermal/Thermal Elements/Thermal Reference
  Conn1 : PMIOPort  Side=Left
  wires:
  T_ENV/1 -> Sum/1
  Constant2/1 -> Sum/2
  Sum/1 -> Simulink-PS Converter1/1
  connections:
  Controlled Temperature Source/LConn1 -- Conn1/RConn1
  Simulink-PS Converter1/RConn1 -- Controlled Temperature Source/RConn1
  Thermal Reference1/LConn1 -- Controlled Temperature Source/RConn2

== system Task_No6/sub_House/Living room/Living Room/Outside Temperature ==
  T_OUT : Inport
  Constant2 : Constant  Value=Conv_C_to_K
  Controlled Temperature Source : fl_lib/Thermal/Thermal Sources/Controlled Temperature Source
  Simulink-PS Converter1 : nesl_utility/Simulink-PS Converter  PhysicalDomain=network_engine_domain  SubClassName=ps_input  LeftPortType=input  RightPortType=output  PseudoPeriodic=off  Frequencies=[]  NoiseDistribution=none  NoiseParameters=[]  Unit=1  AffineConversion=off  FilteringAndDerivatives=provide  SimscapeFilterOrder=1  InputFilterTimeConstant=0.001  UdotUserProvided=0
  Sum : Sum  Inputs=|++
  Thermal Reference1 : fl_lib/Thermal/Thermal Elements/Thermal Reference
  Conn1 : PMIOPort  Side=Left
  wires:
  Sum/1 -> Simulink-PS Converter1/1
  Constant2/1 -> Sum/2
  T_OUT/1 -> Sum/1
  connections:
  Thermal Reference1/LConn1 -- Controlled Temperature Source/RConn2
  Simulink-PS Converter1/RConn1 -- Controlled Temperature Source/RConn1
  Controlled Temperature Source/LConn1 -- Conn1/RConn1

== system Task_No6/sub_House/Living room/Living Room/SOLAR__WALL ==
  Constant : Constant  Value=P_AREA_SOUTH_WALL_LVR
  Constant1 : Constant  Value=P_EM_WALL
  Controlled Heat Flow Rate Source : fl_lib/Thermal/Thermal Sources/Controlled Heat Flow Rate Source
  Product : Product  Inputs=3
  Simulink-PS Converter : nesl_utility/Simulink-PS Converter  PhysicalDomain=network_engine_domain  SubClassName=ps_input  LeftPortType=input  RightPortType=output  PseudoPeriodic=off  Frequencies=[]  NoiseDistribution=none  NoiseParameters=[]  Unit=1  AffineConversion=off  FilteringAndDerivatives=provide  SimscapeFilterOrder=1  InputFilterTimeConstant=0.001  UdotUserProvided=0
  Thermal Reference : fl_lib/Thermal/Thermal Elements/Thermal Reference
  Conn1 : PMIOPort  Side=Left
  wires:
  Constant/1 -> Product/2
  Constant1/1 -> Product/1
  [SOL_SOUTH] -> Product/3
  Product/1 -> Simulink-PS Converter/1
  connections:
  Controlled Heat Flow Rate Source/LConn1 -- Conn1/RConn1
  Simulink-PS Converter/RConn1 -- Controlled Heat Flow Rate Source/RConn1
  Thermal Reference/LConn1 -- Controlled Heat Flow Rate Source/RConn2

== system Task_No6/sub_House/Living room/Living Room/SOLAR__WINDOW ==
  Constant : Constant  Value=P_AREA_WIN_LVR
  Constant1 : Constant  Value=P_EM_GLASS
  Controlled Heat Flow Rate Source : fl_lib/Thermal/Thermal Sources/Controlled Heat Flow Rate Source
  Product : Product  Inputs=3
  Simulink-PS Converter : nesl_utility/Simulink-PS Converter  PhysicalDomain=network_engine_domain  SubClassName=ps_input  LeftPortType=input  RightPortType=output  PseudoPeriodic=off  Frequencies=[]  NoiseDistribution=none  NoiseParameters=[]  Unit=1  AffineConversion=off  FilteringAndDerivatives=provide  SimscapeFilterOrder=1  InputFilterTimeConstant=0.001  UdotUserProvided=0
  Thermal Reference : fl_lib/Thermal/Thermal Elements/Thermal Reference
  Conn1 : PMIOPort  Side=Left
  wires:
  Product/1 -> Simulink-PS Converter/1
  [SOL_SOUTH] -> Product/3
  Constant1/1 -> Product/1
  Constant/1 -> Product/2
  connections:
  Thermal Reference/LConn1 -- Controlled Heat Flow Rate Source/RConn2
  Simulink-PS Converter/RConn1 -- Controlled Heat Flow Rate Source/RConn1
  Controlled Heat Flow Rate Source/LConn1 -- Conn1/RConn1

== system Task_No6/sub_House/Living room/Living Room/TEMP_01 ==
  Constant2 : Constant  Value=Conv_C_to_K
  PS-Simulink Converter : nesl_utility/PS-Simulink Converter  PhysicalDomain=network_engine_domain  SubClassName=ps_output  LeftPortType=input  RightPortType=output  PseudoPeriodic=off  Frequencies=[]  VectorFormat=inherit  Unit=inherit  AffineConversion=off
  Sum : Sum  Inputs=|+-
  Temperature Sensor : fl_lib/Thermal/Thermal Sensors/Temperature Sensor  temperature_measure=foundation.enum.MeasurementReference.difference
  Thermal Reference2 : fl_lib/Thermal/Thermal Elements/Thermal Reference
  PS : PMIOPort  Side=Left
  Sim : Outport
  wires:
  Constant2/1 -> Sum/2
  PS-Simulink Converter/1 -> Sum/1
  Sum/1 -> Sim/1
  connections:
  PS/RConn1 -- Temperature Sensor/LConn1
  PS-Simulink Converter/LConn1 -- Temperature Sensor/RConn2
  Thermal Reference2/LConn1 -- Temperature Sensor/RConn1

== system Task_No6/sub_House/Living room/Living Room/Wall (LVR<->Outside) ==
  InAir-Wall : fl_lib/Thermal/Thermal Elements/Thermal Resistance  resistance=1/(U_WALL*P_AREA_OUTER_WALL_LVR)/2 K/W  T_specify=off  T_priority=None  T=0 K  T_nominal_specify=off  T_nominal_unit=K  T_nominal_value=1  Q_specify=off  Q_priority=None  Q=0 W  Q_nominal_specify=off  Q_nominal_unit=W  Q_nominal_value=1
  Thermal Mass of wall : fl_lib/Thermal/Thermal Elements/Thermal Mass  mass_type=foundation.enum.constant_variable.constant  mass=P_AREA_OUTER_WALL_LVR*(P_THICK_BRICK*P_DENSITY_BRICK+P_THICK_PUR*P_DENSITY_PUR) kg  sp_heat=P_CP_WALL J/(K*kg)  mass_min=1e-6 kg  num_ports=foundation.enum.numPorts2.one  m_specify=off  m_priority=High  m=1 kg  m_nominal_specify=off  m_nominal_unit=kg  m_nominal_value=1  T_specify=on  T_priority=High  T=T_INIT_BDR degC  T_nominal_specify=off  T_nominal_unit=K  T_nominal_value=1  Q_specify=off  Q_priority=None  Q=0 W  Q_nominal_specify=off  Q_nominal_unit=W  Q_nominal_value=1
  Wall-OutAir : fl_lib/Thermal/Thermal Elements/Thermal Resistance  resistance=1/(U_WALL*P_AREA_OUTER_WALL_LVR)/2 K/W  T_specify=off  T_priority=None  T=0 K  T_nominal_specify=off  T_nominal_unit=K  T_nominal_value=1  Q_specify=off  Q_priority=None  Q=0 W  Q_nominal_specify=off  Q_nominal_unit=W  Q_nominal_value=1
  Conn1 : PMIOPort  Side=Left
  Conn3 : PMIOPort  Port=2  Side=Right
  Conn2 : PMIOPort  Port=3  Side=Right
  connections:
  Wall-OutAir/RConn1 -- Conn2/RConn1
  Wall-OutAir/LConn1 -- Conn3/RConn1 -- Thermal Mass of wall/LConn1 -- InAir-Wall/RConn1
  Conn1/RConn1 -- InAir-Wall/LConn1

== system Task_No6/sub_House/Living room/Living Room/Window (LVR<->Outside) ==
  InAir-Window : fl_lib/Thermal/Thermal Elements/Thermal Resistance  resistance=1/(U_WINDOW*P_AREA_WIN_LVR)/2 K/W  T_specify=off  T_priority=None  T=0 K  T_nominal_specify=off  T_nominal_unit=K  T_nominal_value=1  Q_specify=off  Q_priority=None  Q=0 W  Q_nominal_specify=off  Q_nominal_unit=W  Q_nominal_value=1
  Thermal Mass of window : fl_lib/Thermal/Thermal Elements/Thermal Mass  mass_type=foundation.enum.constant_variable.constant  mass=P_M_WINDOW_SPEC*P_AREA_WIN_LVR kg  sp_heat=P_CP_GLASS J/(K*kg)  mass_min=1e-6 kg  num_ports=foundation.enum.numPorts2.one  m_specify=off  m_priority=High  m=1 kg  m_nominal_specify=off  m_nominal_unit=kg  m_nominal_value=1  T_specify=on  T_priority=High  T=T_INIT_BDR degC  T_nominal_specify=off  T_nominal_unit=K  T_nominal_value=1  Q_specify=off  Q_priority=None  Q=0 W  Q_nominal_specify=off  Q_nominal_unit=W  Q_nominal_value=1
  Window-OutAir : fl_lib/Thermal/Thermal Elements/Thermal Resistance  resistance=1/(U_WINDOW*P_AREA_WIN_LVR)/2 K/W  T_specify=off  T_priority=None  T=0 K  T_nominal_specify=off  T_nominal_unit=K  T_nominal_value=1  Q_specify=off  Q_priority=None  Q=0 W  Q_nominal_specify=off  Q_nominal_unit=W  Q_nominal_value=1
  Conn1 : PMIOPort  Side=Right
  Conn2 : PMIOPort  Port=2  Side=Left
  Conn3 : PMIOPort  Port=3  Side=Right
  connections:
  Conn2/RConn1 -- InAir-Window/LConn1
  Conn1/RConn1 -- Window-OutAir/RConn1
  InAir-Window/RConn1 -- Conn3/RConn1 -- Thermal Mass of window/LConn1 -- Window-OutAir/LConn1

== system Task_No6/sub_House/Living room/MA Living Room/Environment_in ==
  Constant1 : Constant  Value=P_INIT_CO2
  Constant4 : Constant  Value=1e5
  Constant6 : Constant  Value=Conv_C_to_K
  Controlled Reservoir (MA) : fl_lib/Moist Air/Elements/Controlled Reservoir (MA)  moisture_spec=foundation.enum.moistureSpec.RelativeHumidity  trace_gas_spec=foundation.enum.trace_gas_spec.mass_fraction  RH_ws=1  area_A=P_AREA_DUCT m^2  input_error_spec=foundation.enum.input_range_error.warn
      settings: InternalSimscapePortConfiguration="{\"Bottom\":[],\"Left\":[{\"id\":\"A\",\"label\":\"A\",\"type\":\"foundation.moist_air.moist_air\"}],\"Right\":[{\"id\":\"T\",\"label\":\"T\",\"type\":\"input\"},{\"id\":\"P\",\"label\":\"P\",\"type\":\"input\"},{\"id\":\"W\",\"label\":\"W\",\"type\":\"input\"},{\"id\":\"G\",\"label\":\"G\",\"type\":\"input\"}],\"Top\":[]}"
  Gain : Gain  Gain=1/100
  Gain2 : Gain  Gain=1e-6
  Simulink-PS Converter{3,5..7} (4 alike) : nesl_utility/Simulink-PS Converter  PhysicalDomain=network_engine_domain  SubClassName=ps_input  LeftPortType=input  RightPortType=output  PseudoPeriodic=off  Frequencies=[]  NoiseDistribution=none  NoiseParameters=[]  Unit=1  AffineConversion=off  FilteringAndDerivatives=provide  SimscapeFilterOrder=1  InputFilterTimeConstant=0.001  UdotUserProvided=0
  Sum2 : Sum  Inputs=|++
  Conn1 : PMIOPort  Side=Left
  wires:
  Constant1/1 -> Gain2/1
  Constant6/1 -> Sum2/2
  Gain/1 -> Simulink-PS Converter6/1
  Constant4/1 -> Simulink-PS Converter5/1
  Gain2/1 -> Simulink-PS Converter7/1
  Sum2/1 -> Simulink-PS Converter3/1
  [T_OUT] -> Sum2/1
  [RH_OUT] -> Gain/1
  connections:
  Simulink-PS Converter3/RConn1 -- Controlled Reservoir (MA)/RConn1
  Simulink-PS Converter7/RConn1 -- Controlled Reservoir (MA)/RConn4
  Controlled Reservoir (MA)/LConn1 -- Conn1/RConn1
  Simulink-PS Converter5/RConn1 -- Controlled Reservoir (MA)/RConn2
  Simulink-PS Converter6/RConn1 -- Controlled Reservoir (MA)/RConn3
